simulink model "Robust_Control"  (R2023a)
settings: Solver=VariableStepAuto  StartTime=0.0  StopTime=30  RelTol=1e-3
model workspace: external: MAT-File (data not in the file)
undefined symbols (not defined in the file): D, DiscIntNeverNeededParam, f_s, Kd_r, Kp_r, Q
settings Model: Creator=benit  LastModifiedBy=Savio Del Peschio
settings OptimizationCC: ReuseModelBlockBuffer=off

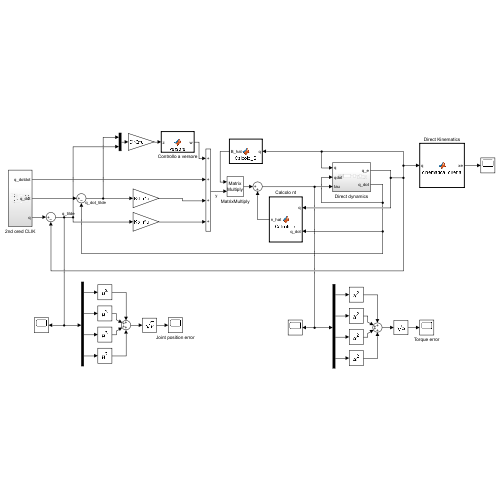
[thumbnail: Simulink's stored preview of the top-level diagram]
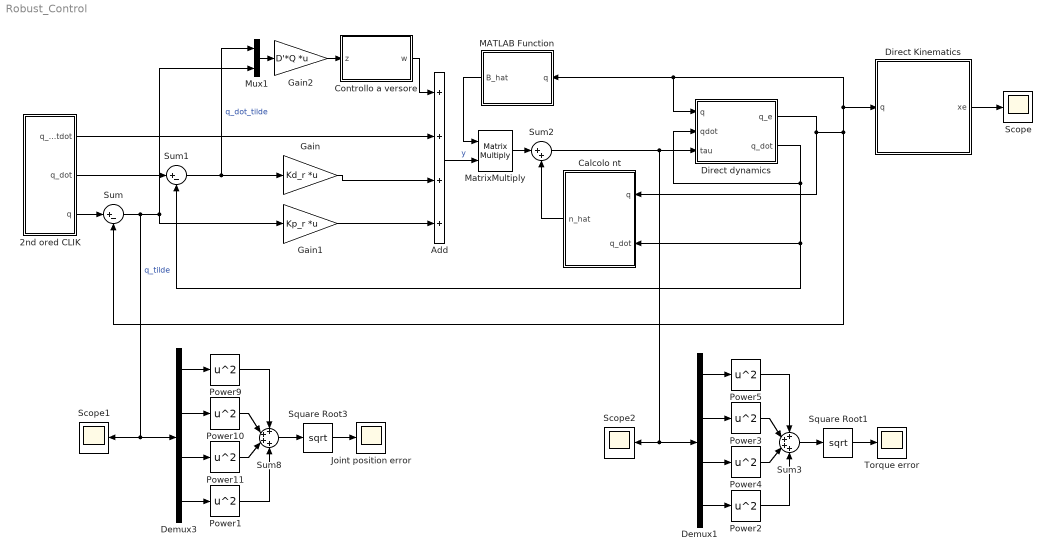
== system Robust_Control ==
  2nd ored CLIK : Subsystem
  Add : Sum  Inputs=++++
  Calcolo nt : MATLAB Function  TreatAsAtomicUnit=on
  Controllo a versore : MATLAB Function  TreatAsAtomicUnit=on
  Demux1 : Demux
  Demux3 : Demux
  Direct Kinematics : MATLAB Function  TreatAsAtomicUnit=on
  Direct dynamics : Subsystem
  Gain : Gain  Gain=Kd_r  Multiplication=Matrix(K*u)
  Gain1 : Gain  Gain=Kp_r  Multiplication=Matrix(K*u)
  Gain2 : Gain  Gain=D'*Q  Multiplication=Matrix(K*u)
  Joint position error : Scope
  MATLAB Function : MATLAB Function  TreatAsAtomicUnit=on
  MatrixMultiply : Product  Multiplication=Matrix(*)
  Mux1 : Mux  Inputs=2
  Power{1..5,9..11} (8 alike) : Math  Operator=square
  Scope : Scope
  Scope1 : Scope
  Scope2 : Scope
  Square Root1 : Sqrt
  Square Root3 : Sqrt
  Sum : Sum  Inputs=|+-
  Sum1 : Sum  Inputs=|+-
  Sum2 : Sum  Inputs=|++
  Sum3 : Sum  Inputs=++++
  Sum8 : Sum  Inputs=++++
  Torque error : Scope
  wires:
  2nd ored CLIK/2(q_dot) -> Sum1/1
  Sum1/1 -> Gain/1, Mux1/1  "q_dot_tilde"
  Sum/1 -> Scope1/1, Demux3/1, Gain1/1, Mux1/2  "q_tilde"
  Gain/1 -> Add/3
  Gain2/1 -> Controllo a versore/1(z)
  Controllo a versore/1(w) -> Add/1
  Mux1/1 -> Gain2/1
  MATLAB Function/1(B_hat) -> MatrixMultiply/1
  Add/1 -> MatrixMultiply/2  "y"
  MatrixMultiply/1 -> Sum2/1
  Calcolo nt/1(n_hat) -> Sum2/2
  Direct dynamics/1(q_e) -> Direct Kinematics/1(q), Direct dynamics/1(q), MATLAB Function/1(q), Sum/2, Calcolo nt/1(q)
  Direct dynamics/2(q_dot) -> Calcolo nt/2(q_dot), Sum1/2, Direct dynamics/2(qdot)
  Direct Kinematics/1(xe) -> Scope/1
  Demux3/2 -> Power10/1
  Square Root3/1 -> Joint position error/1
  Demux3/4 -> Power1/1
  Power11/1 -> Sum8/3
  Power1/1 -> Sum8/4
  Demux3/1 -> Power9/1
  Power9/1 -> Sum8/1
  Sum8/1 -> Square Root3/1
  Demux3/3 -> Power11/1
  Power10/1 -> Sum8/2
  Sum2/1 -> Scope2/1, Demux1/1, Direct dynamics/3(tau)
  2nd ored CLIK/1(q_dotdot) -> Add/2
  2nd ored CLIK/3(q) -> Sum/1
  Gain1/1 -> Add/4
  Demux1/1 -> Power5/1
  Demux1/3 -> Power4/1
  Power3/1 -> Sum3/2
  Sum3/1 -> Square Root1/1
  Demux1/2 -> Power3/1
  Power4/1 -> Sum3/3
  Power5/1 -> Sum3/1
  Power2/1 -> Sum3/4
  Demux1/4 -> Power2/1
  Square Root1/1 -> Torque error/1

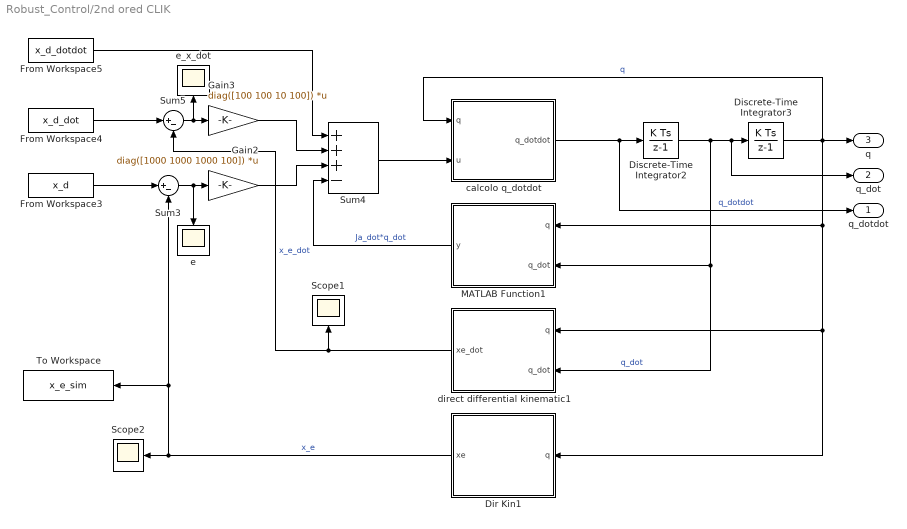
== system Robust_Control/2nd ored CLIK ==
  Dir Kin1 : MATLAB Function  TreatAsAtomicUnit=on
  Discrete-Time Integrator2 : DiscreteIntegrator  gainval=1  InitialCondition=zeros(4,1)  SampleTime=1/f_s  ICPrevOutput=DiscIntNeverNeededParam  ICPrevScaledInput=DiscIntNeverNeededParam
  Discrete-Time Integrator3 : DiscreteIntegrator  gainval=1  InitialCondition=config_p_init'  SampleTime=1/f_s  ICPrevOutput=DiscIntNeverNeededParam  ICPrevScaledInput=DiscIntNeverNeededParam
  From Workspace3 : FromWorkspace  VariableName=x_d
  From Workspace4 : FromWorkspace  VariableName=x_d_dot
  From Workspace5 : FromWorkspace  VariableName=x_d_dotdot
  Gain2 : Gain  Gain=diag([1000 1000 1000 100])  Multiplication=Matrix(K*u)
  Gain3 : Gain  Gain=diag([100 100 10 100])  Multiplication=Matrix(K*u)
  MATLAB Function1 : MATLAB Function  TreatAsAtomicUnit=on
  Scope1 : Scope
  Scope2 : Scope
  Sum3 : Sum  Inputs=|+-
  Sum4 : Sum  Inputs=+++-
  Sum5 : Sum  Inputs=|+-
  To Workspace : ToWorkspace  VariableName=x_e_sim  SaveFormat=Timeseries  SampleTime=-1
  calcolo q_dotdot : MATLAB Function  TreatAsAtomicUnit=on
  direct differential kinematic1 : MATLAB Function  TreatAsAtomicUnit=on
  e : Scope
  e_x_dot : Scope
  q_dotdot : Outport
  q_dot : Outport  Port=2
  q : Outport  Port=3
  wires:
  Gain3/1 -> Sum4/2
  Sum5/1 -> e_x_dot/1, Gain3/1
  direct differential kinematic1/1(xe_dot) -> Sum5/2, Scope1/1  "x_e_dot"
  Gain2/1 -> Sum4/3
  From Workspace4/1 -> Sum5/1
  calcolo q_dotdot/1(q_dotdot) -> q_dotdot/1, Discrete-Time Integrator2/1  "q_dotdot"
  From Workspace5/1 -> Sum4/1
  From Workspace3/1 -> Sum3/1
  MATLAB Function1/1(y) -> Sum4/4  "Ja_dot*q_dot"
  Sum3/1 -> e/1, Gain2/1
  Dir Kin1/1(xe) -> To Workspace/1, Sum3/2, Scope2/1  "x_e"
  Discrete-Time Integrator2/1 -> direct differential kinematic1/2(q_dot), MATLAB Function1/2(q_dot), q_dot/1, Discrete-Time Integrator3/1  "q_dot"
  Discrete-Time Integrator3/1 -> q/1, Dir Kin1/1(q), direct differential kinematic1/1(q), MATLAB Function1/1(q), calcolo q_dotdot/1(q)  "q"
  Sum4/1 -> calcolo q_dotdot/2(u)

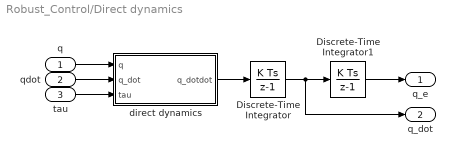
== system Robust_Control/Direct dynamics ==
  q : Inport
  qdot : Inport  Port=2
  tau : Inport  Port=3
  Discrete-Time Integrator : DiscreteIntegrator  InitialCondition=zeros(4,1)  SampleTime=1/f_s  ICPrevOutput=DiscIntNeverNeededParam  ICPrevScaledInput=DiscIntNeverNeededParam
  Discrete-Time Integrator1 : DiscreteIntegrator  InitialCondition=config_p_init'  SampleTime=1/f_s  ICPrevOutput=DiscIntNeverNeededParam  ICPrevScaledInput=DiscIntNeverNeededParam
  direct dynamics : MATLAB Function  TreatAsAtomicUnit=on
  q_e : Outport
  q_dot : Outport  Port=2
  wires:
  direct dynamics/1(q_dotdot) -> Discrete-Time Integrator/1
  qdot/1 -> direct dynamics/2(q_dot)
  Discrete-Time Integrator/1 -> q_dot/1, Discrete-Time Integrator1/1
  tau/1 -> direct dynamics/3(tau)
  q/1 -> direct dynamics/1(q)
  Discrete-Time Integrator1/1 -> q_e/1

== matlab function Robust_Control/Controllo a versore ==
  data: z input; w output
function w = versore(z)
    rho=50; 
    epsilon=0.2;
     
    if norm(z) < epsilon
        w=rho*z / epsilon;
    else
        w=rho*z / norm(z);
    end
end

== matlab function Robust_Control/MATLAB Function ==
  data: q input; B_hat output
function B_hat= Calcolo_B(q)

    B_hat=diag([10*cos(q(2)) + 10763/500, 4383/500, 45/2, 7/5]);

end

== matlab function Robust_Control/Direct dynamics/direct dynamics ==
  data: q input; q_dot input; q_dotdot output; tau input
function q_dotdot = fcn(q, q_dot, tau)
       
    %attriti dei motori
    Fm1 = 0.00005;
    Fm2 = 0.00005;
    Fm3 = 0.01;
    Fm4 = 0.005;
    
    theta_2 = q(2);
    theta_dot_1 = q_dot(1);
    theta_dot_2 = q_dot(2);
    d_dot_3 = q_dot(3);
    theta_dot_4 = q_dot(4);
    
    B_p = [(25*cos(theta_2))/2 + 12013/500, (25*cos(theta_2))/4 + 1252/125, -1/4, -51/50;
            (25*cos(theta_2))/4 + 1252/125,                       1252/125, -1/4, -51/50;
                                      -1/4,                           -1/4, 55/2,      0;
                                    -51/50,                         -51/50,    0,    7/5];                                                                                                        
       
    C_p = [-(25*theta_dot_2*sin(theta_2))/4, - (25*theta_dot_1*sin(theta_2))/4 - (25*theta_dot_2*sin(theta_2))/4, 0, 0;
            (25*theta_dot_1*sin(theta_2))/4,                                                                   0, 0, 0;
                                          0,                                                                   0, 0, 0;
                                          0,                                                                   0, 0, 0];
    
    
    Fv = diag([-Fm1 -Fm2 -Fm3 -Fm4]);
    g = [0, 0, - 9.81*(5+10), 0]';
    tau_primo = C_p*q_dot+Fv*q_dot+g;
    
    q_dotdot = inv(B_p)*(tau-tau_primo); 

end

== matlab function Robust_Control/Calcolo nt ==
  data: q input size=[4]; q_dot input; n_hat output
function n_hat = Calcolo_n(q, q_dot)
    
    % attriti dei motori
    Fm1 = 0.00005;
    Fm2 = 0.00005;
    Fm3 = 0.01;
    Fm4 = 0.005;
    
    theta_1 = q(1);
    theta_2 = q(2);
    d_3 = q(3);
    theta_4 = q(4);
    theta_dot_1 = q_dot(1);
    theta_dot_2 = q_dot(2);
    
    C = [-5*theta_dot_2*sin(theta_2), -5*theta_dot_1*sin(theta_2) - 5*theta_dot_2*sin(theta_2), 0, 0;
          5*theta_dot_1*sin(theta_2), 0,                                                        0, 0;
          0,                          0,                                                        0, 0;
          0,                          0,                                                        0, 0];
    
    Fv = diag([-Fm1 -Fm2 -Fm3 -Fm4]);
    
    g = [0, 0, -9.81*10, 0]';
    
    n_hat= C*q_dot+Fv*q_dot+g;

    
end

== matlab function Robust_Control/Direct Kinematics ==
  data: q input; xe output
function xe = cinematica_diretta(q)
    
    xe = [  0.5*cos(q(1))+0.5*cos(q(1)+q(2));
            0.5*sin(q(1))+0.5*sin(q(1)+q(2));
            1/2-q(3)
            q(1)+q(2)-q(4) ];

end

== matlab function Robust_Control/2nd ored CLIK/Dir Kin1 ==
  data: q input; xe output
function xe = cinematica_diretta(q)
    
    xe = [  0.5*cos(q(1))+0.5*cos(q(1)+q(2));
            0.5*sin(q(1))+0.5*sin(q(1)+q(2));
            1/2-q(3)
            q(1)+q(2)-q(4) ];

end

== matlab function Robust_Control/2nd ored CLIK/MATLAB Function1 ==
  data: q input; q_dot input; y output
function y = Ja_dot(q, q_dot)

    J_min_dot = [-0.5*(q_dot(1)+q_dot(2))*cos(q(1)+q(2))-0.5*q_dot(1)*cos(q(1))              -0.5*(q_dot(1)+q_dot(2))*cos(q(1)+q(2))  0   0
                 -0.5*(q_dot(1)+q_dot(2))*sin(q(1)+q(2))-0.5*q_dot(1)*sin(q(1))              -0.5*(q_dot(1)+q_dot(2))*sin(q(1)+q(2))  0   0
                 0                                                                            0                                       0   0
                 0                                                                            0                                       0   0];
    
     y = J_min_dot*q_dot;
     
end

== matlab function Robust_Control/2nd ored CLIK/calcolo q_dotdot ==
  data: q input; u input; q_dotdot output
function q_dotdot = fcn(q,u)

    J = [-0.5*sin(q(1))-0.5*sin(q(1)+q(2))   -0.5*sin(q(1)+q(2))    0  0 
          0.5*cos(q(1))+0.5*cos(q(1)+q(2))    0.5*cos(q(1)+q(2))    0  0 
          0                                   0                    -1  0
          1                                   1                     0  -1];
    
    q_dotdot = pinv(J)*u;

end

== matlab function Robust_Control/2nd ored CLIK/direct differential kinematic1 ==
  data: q input; q_dot input; xe_dot output
function xe_dot = fcn(q,q_dot)

 Ja = [-0.5*sin(q(1))-0.5*sin(q(1)+q(2)) -0.5*sin(q(1)+q(2))    0 0
      0.5*cos(q(1))+0.5*cos(q(1)+q(2))  0.5*cos(q(1)+q(2))     0 0
      0                                0                    -1 0
      1                                1                    0 -1];

xe_dot = Ja*q_dot;

end
